simulink model "distributed_project_square"  (R2025b)
settings: Solver=VariableStepAuto  StartTime=0.0  StopTime=10  RelTol=1e-3  AbsTol=1e-3  EnableMultiTasking=on
model workspace (MAT data in the model file):
  t_now = 10
  v = 1
values from neighbouring files (symbols this model uses):
  m = 20    [FirstRegression.m]
  msg_init =     [distributed_project_adjusted.mat]
  N = min([length(e1), length(e2), length(e3), N_max])    [10_runs_result_for_odometer.m]    (also in cc.m = min(length(e1), length(e2)); distributed_project_adjusted.mat = 100; distributed_stats.m = min([length(e1),length(e2),length(e3)]); ten_runs_result_for_odometer.m)
  r = 0.05    [distributed_project.mat]    (also in distributed_project_adjusted.mat)
undefined symbols (not defined in the file or in its folder): fractalcoef, X, Y, Z
libraries: nesl_utility x69, sm_lib x50, simulink x20, matrix_library x20, mspfiltlib x4, sensorgpslib x4, mspsensorlib x4
(part 4 of 5)

== matlab function distributed_project_square/MATLAB Function1 ==
  data: x output; lat input; y output; lon input
function [x,y] = getXY(lat, lon)

% Reference point
persistent lat0 lon0 initialized

if isempty(initialized)
    lat0 = lat;
    lon0 = lon;
    initialized = true;
end



% Convert to radians
lat0_rad = deg2rad(lat0);
lon0_rad = deg2rad(lon0);
lat_rad  = deg2rad(lat);
lon_rad  = deg2rad(lon);

% Earth radius
R = 6371000; % meters

% Compute local x, y
lat_avg = (lat_rad + lat0_rad)/2;
x = R * (lon_rad - lon0_rad) * cos(lat_avg); % east
y = R * (lat_rad - lat0_rad);                 % north

== matlab function distributed_project_square/MATLAB Function2 ==
  data: msg_in input; x_hat_neighbors output; neighbor_idx output; P_j_neighbours output; N output; my_id input; t_now input size=1
function [x_hat_neighbors, neighbor_idx, P_j_neighbours, N] = ...
         receive_msg(msg_in, my_id, t_now)
%#codegen

%% Fixed dimensions — must be constants for codegen
MAX_AGENTS  = 7;
STATE_DIM   = 5;
P_DIM       = 5;
T_WINDOW    = 5.0;   % seconds — max message age

N = 0;

for i = 1:length(msg_in)
    if msg_in(i).ID ~= 0   % assume ID=0 means empty slot
        N = N + 1;
    end
end


%% Fixed-size outputs — codegen requires known dimensions
x_hat_neighbors = zeros(STATE_DIM, MAX_AGENTS);
P_j_neighbours  = zeros(P_DIM, P_DIM, MAX_AGENTS);
neighbor_idx    = zeros(1, MAX_AGENTS);
N_neighbors     = 0;




%% Persistent store — holds latest message per agent slot
%% Indexed by agent ID (1..MAX_AGENTS)
persistent latest_x latest_P latest_t latest_valid

if isempty(latest_x)
    latest_x     = zeros(STATE_DIM, MAX_AGENTS);
    latest_P     = zeros(P_DIM, P_DIM, MAX_AGENTS);
    latest_t     = -inf(1, MAX_AGENTS);   % never received
    latest_valid = zeros(1, MAX_AGENTS);  % 0 = no data
end

%% ── Step 1: Update persistent store with incoming messages ────────
for k = 1:length(msg_in)
    id = msg_in(k).ID;

    %% Skip invalid IDs
    if id < 1 || id > N
        continue;
    end

    %% Skip own messages
    if id == my_id
        continue;
    end

    %% Keep only the latest message per ID
    if msg_in(k).t > latest_t(id)
        latest_x(:, id)      = msg_in(k).x;
        latest_P(:, :, id)   = msg_in(k).P;
        latest_t(id)         = msg_in(k).t;
        latest_valid(id)     = 1;
    end
end

%% ── Step 2: Collect valid neighbours within time window ───────────
for id = 1:N

    %% Skip self
    if id == my_id
        continue;
    end

    %% Skip slots never received
    if latest_valid(id) == 0
        continue;
    end

    %% Skip stale messages
    msg_age = t_now - latest_t(id);
    if msg_age > T_WINDOW || msg_age < 0
        continue;
    end

    %% Valid neighbour — add to output
    N_neighbors = N_neighbors + 1;
    x_hat_neighbors(:, N_neighbors) = latest_x(:, id);
    P_j_neighbours(:,:, N_neighbors) = latest_P(:,:, id);
    neighbor_idx(N_neighbors) = id;
end





end

== matlab function distributed_project_square/Subsystem2/MATLAB Function8 ==
  data: N_i input; N_final output; trigger output
function [N_final, trigger] = convergence_detector(N_i)

%#codegen

% PARAMETERS
k = 5;   % number of steps for stability

% PERSISTENT MEMORY
persistent buffer count

    if isempty(buffer)
        buffer = zeros(k,1);
        count = 0;
    end

% SHIFT BUFFER (like Unit Delay chain)
buffer = [buffer(2:end); N_i];

% CHECK IF ALL VALUES SAME


    if all(buffer == buffer(1))
        count = count + 1;
    else
        count = 0;
    end

    % TRIGGER WHEN STABLE
    if count >= 1   % already stable for k steps
        trigger = 1;
        N_final = buffer(end);
    else
        trigger = 0;
        N_final = N_i;
    end

end

== matlab function distributed_project_square/MATLAB Function4 ==
  data: ID_i input; delta_i output double; N input; formation input
function delta_i = formation_calculator(ID_i, N, formation)
    %#codegen
    
    delta_i = [0; 0];
    
    if N <= 0 || ID_i < 1 || ID_i > N || N == 1
        return;
    end
    spacing = 1.5;
    switch formation
        case 1  % LINE (N ≤ 2)
            center = (N - 1) / 2;
            delta_i = double([(ID_i - 1 - center) * spacing; 0]);
            
        case 2  % CIRCLE (N ≥ 5)
            radius = spacing * N / (2 * pi);
            theta = 2 * pi * (ID_i - 1) / N;
            delta_i = radius * [cos(double(theta)); sin(double(theta))];
            
        case 3  % SQUARE (N = 4)
            half = spacing / 2;
            corners = [ half, -half, -half,  half;   % x-coordinates
                       -half, -half,  half,  half];  % y-coordinates
            delta_i = corners(:, ID_i);
            
        case 4  % TRIANGLE (N = 3)
            side = spacing * 2;
            h = sqrt(3) / 2 * side;
            vertices = [0,   -side/2,  side/2;    % x-coordinates
                       2*h/3, -h/3,   -h/3];     % y-coordinates
            delta_i = vertices(:, ID_i);
            
        otherwise
            delta_i = [0; 0];
    end
end

== matlab function distributed_project_square/MATLAB Function5 ==
  data: N_final input; formation output
function formation = formation_selector(N_final)


    if N_final <= 0
        formation = 0;  % Invalid
        warning('Invalid number of agents: %d', N_final);
        return;
    end

    if N_final <= 2
        formation = 1;
    elseif N_final == 3
        formation = 4;
    elseif N_final == 4
        formation = 3;
    else
        formation = 2;
    end

end

== matlab function distributed_project_square/MATLAB Function6 ==
  data: x_fused input; ei_pos_f output; x_c input; delta_i input; ei_norm output; x_c_raw input
function [ei_pos_f, ei_norm] = formation_error_calculator(...
                               x_fused, x_c, delta_i, x_c_raw)
%#codegen
persistent ei_prev;
if isempty(ei_prev)
    ei_prev = zeros(2,1);
end
ei_pos_raw = (x_c + delta_i) - x_fused(1:2);

%% Low-pass filter — smooth noise
alpha    = 0.167;   % Ts=0.01, tau=0.05s
ei_pos_f = (1-alpha)*ei_prev + alpha*ei_pos_raw;

%% Use raw norm for threshold (not filtered)
ei_norm = norm((x_c_raw + delta_i) - x_fused(1:2));
ei_prev = ei_pos_f;
end

== matlab function distributed_project_square/MATLAB Function7 ==
  data: ei_pos input; ei_vel input; kp input; kd input; L input; vL output size=1; vR output size=1; theta input; w_scaled output; u output
function [vL, vR, w_scaled, u] = control_law(ei_pos, ei_vel, kp, kd, L, theta)
%#codegen

u = [0.0; 0.0];
w_scaled = double(0);
vL = double(0);
vR = double(0);

%% Deadband for spacing=0.3m
e_dead = 0.08;
if norm(ei_pos) < e_dead
    return;
end

u = kp * ei_pos - kd * ei_vel;

%% Tighter saturation for small formation
u_max  = 0.4;
u_norm = sqrt(u(1)^2 + u(2)^2);
if u_norm > u_max
    u = u * (u_max / u_norm);
end

v_lin =  cos(theta)*u(1) + sin(theta)*u(2);
w     = -sin(theta)*u(1) + cos(theta)*u(2);

w_scaled = w / (L/2);

v_max = 0.4;     % slower for small formation
w_max = 0.4;
v_lin    = max(-v_max, min(v_max, v_lin));
w_scaled = max(-w_max, min(w_max, w_scaled));

vL = v_lin - (L/2)*w_scaled;
vR = v_lin + (L/2)*w_scaled;
end

== matlab function distributed_project_square/Subsystem/MATLAB Function1 ==
  data: pos_x input; x_next output; pos_y input; theta input; v input; a input; w input; P_next output; gyro_bias input
function [x_next, P_next] = local_ekf_predict(pos_x,pos_y, theta, v, a, w, gyro_bias)
% MOTION_UPDATE: Predicts the next state and covariance for a 2D vehicle
%
% Inputs:
%   x  - current state [x; y; theta; v]
%   P  - current state covariance (4x4)
%   u  - control input [a; omega] (acceleration, angular rate)
%   Q  - process noise covariance (4x4)
%   dt - time step Δt
%
% Outputs:
%   x_next - predicted next state
%   P_next - predicted next covariance

dt = 0.01;
Q = eye(5)*0.01;
% Make P persistent across calls
persistent P;
    if isempty(P)
        P = eye(5) * 0.1;  % initialize first time
    end

% State prediction (nonlinear)
x_next = zeros(5,1);

              % angular velocity (yaw)
bias_z = gyro_bias(3);      % gyro bias (yaw)
v = norm(v);
a = norm(a);
x_next(1) = pos_x + v * cos(theta) * dt;
x_next(2) = pos_y + v * sin(theta) * dt;
x_next(3) = theta + w * dt;
x_next(4) = v + a * dt;
x_next(5) = bias_z;

% Jacobian F_k = ∂f/∂x
A = [ 1, 0, -v*sin(theta)*dt, cos(theta)*dt, 0;
      0, 1,  v*cos(theta)*dt, sin(theta)*dt, 0;
      0, 0, 1,                 0,            -dt;
      0, 0, 0,                 1,             0;
      0, 0, 0,                 0,             1];

% Covariance prediction
P_next = A * P * A' + Q;
P = P_next;
end

== matlab function distributed_project_square/MATLAB Function10 ==
  data: quat input; theta output
function theta = quat_to_angle(quat)
%#codegen

% normalize (important if coming from simulation)
quat = quat / norm(quat);

w = quat(1);
z = quat(4);

theta = 2 * atan2(z, w);

end

== matlab function distributed_project_square/MATLAB Function11 ==
  data: x output; lat input; y output; lon input
function [x,y] = getXY(lat, lon)

% Reference point
persistent lat0 lon0 initialized

if isempty(initialized)
    lat0 = lat;
    lon0 = lon;
    initialized = true;
end



% Convert to radians
lat0_rad = deg2rad(lat0);
lon0_rad = deg2rad(lon0);
lat_rad  = deg2rad(lat);
lon_rad  = deg2rad(lon);

% Earth radius
R = 6371000; % meters

% Compute local x, y
lat_avg = (lat_rad + lat0_rad)/2;
x = R * (lon_rad - lon0_rad) * cos(lat_avg); % east
y = R * (lat_rad - lat0_rad);                 % north

== matlab function distributed_project_square/MATLAB Function12 ==
  data: x_c_raw input; x_c_out output size=[2, 1]; all_converged input; x_c_raw output
function [x_c_out, x_c_raw] = centroid_manager(x_c_raw, all_converged)
%#codegen

persistent x_c_latched is_latched;
if isempty(x_c_latched)
    x_c_latched = zeros(2,1);
    is_latched  = false;
end

if all_converged && ~is_latched
    %% Latch centroid at moment of convergence
    x_c_latched = x_c_raw;
    is_latched  = true;
end

if is_latched
    x_c_out = x_c_latched;
else
    x_c_out = x_c_raw;
end
end

== matlab function distributed_project_square/MATLAB Function13 ==
  data: x_i_cons input; x_hat_neighbors input; N_all input; x_c output
function x_c = centroid_estimator(x_i_cons, x_hat_neighbors, N_all)
%#codegen
%% Inputs:
%%   x_i_cons        - own consensus state  (5×1)
%%   x_hat_neighbors - neighbour states     (5×N_neighbors)
%%                     columns 1..N_neighbors are valid
%%   N_neighbors     - actual neighbour count (not N_max)
%%
%% Output:
%%   x_c             - centroid (2×1)

%% Own position — always (2×1) after explicit indexing
own_pos = [x_i_cons(1); x_i_cons(2)];   % explicit 2×1, no reshape


%% Sum own position
pos_sum = own_pos;

%% Add each neighbour position explicitly
for j = 1:N_all-1
    pos_sum = pos_sum + [x_hat_neighbors(1,j); x_hat_neighbors(2,j)];
end

%% Average over total count
x_c   = pos_sum / N_all;
end

== matlab function distributed_project_square/MATLAB Function14 ==
  data: ID_i input; delta_i output double; N input; formation input
function delta_i = formation_calculator(ID_i, N, formation)
    %#codegen
    
    delta_i = [0; 0];
    
    if N <= 0 || ID_i < 1 || ID_i > N || N == 1
        return;
    end
    spacing = 1.5;
    switch formation
        case 1  % LINE (N ≤ 2)
            center = (N - 1) / 2;
            delta_i = double([(ID_i - 1 - center) * spacing; 0]);
            
        case 2  % CIRCLE (N ≥ 5)
            radius = spacing * N / (2 * pi);
            theta = 2 * pi * (ID_i - 1) / N;
            delta_i = radius * [cos(double(theta)); sin(double(theta))];
            
        case 3  % SQUARE (N = 4)
            half = spacing / 2;
            corners = [ half, -half, -half,  half;   % x-coordinates
                       -half, -half,  half,  half];  % y-coordinates
            delta_i = corners(:, ID_i);
            
        case 4  % TRIANGLE (N = 3)
            side = spacing * 2;
            h = sqrt(3) / 2 * side;
            vertices = [0,   -side/2,  side/2;    % x-coordinates
                       2*h/3, -h/3,   -h/3];     % y-coordinates
            delta_i = vertices(:, ID_i);
            
        otherwise
            delta_i = [0; 0];
    end
end

== matlab function distributed_project_square/MATLAB Function15 ==
  data: N_final input; formation output
function formation = formation_selector(N_final)


    if N_final <= 0
        formation = 0;  % Invalid
        warning('Invalid number of agents: %d', N_final);
        return;
    end

    if N_final <= 2
        formation = 1;
    elseif N_final == 3
        formation = 4;
    elseif N_final == 4
        formation = 3;
    else
        formation = 2;
    end

end

== matlab function distributed_project_square/MATLAB Function17 ==
  data: x_fused input; ei_pos_f output; x_c input; delta_i input; ei_norm output; x_c_raw input
function [ei_pos_f, ei_norm] = formation_error_calculator(...
                               x_fused, x_c, delta_i, x_c_raw)
%#codegen
persistent ei_prev;
if isempty(ei_prev)
    ei_prev = zeros(2,1);
end
ei_pos_raw = (x_c + delta_i) - x_fused(1:2);

%% Low-pass filter — smooth noise
alpha    = 0.167;   % Ts=0.01, tau=0.05s
ei_pos_f = (1-alpha)*ei_prev + alpha*ei_pos_raw;

%% Use raw norm for threshold (not filtered)
ei_norm = norm((x_c_raw + delta_i) - x_fused(1:2));
ei_prev = ei_pos_f;
end

== matlab function distributed_project_square/MATLAB Function18 ==
  data: ei_pos input; ei_vel input; kp input; kd input; L input; vL output size=1; vR output size=1; theta input; w_scaled output; u output
function [vL, vR, w_scaled, u] = control_law(ei_pos, ei_vel, kp, kd, L, theta)
%#codegen

u = [0.0; 0.0];
w_scaled = double(0);
vL = double(0);
vR = double(0);

%% Deadband for spacing=0.3m
e_dead = 0.08;
if norm(ei_pos) < e_dead
    return;
end

u = kp * ei_pos - kd * ei_vel;

%% Tighter saturation for small formation
u_max  = 0.4;
u_norm = sqrt(u(1)^2 + u(2)^2);
if u_norm > u_max
    u = u * (u_max / u_norm);
end

v_lin =  cos(theta)*u(1) + sin(theta)*u(2);
w     = -sin(theta)*u(1) + cos(theta)*u(2);

w_scaled = w / (L/2);

v_max = 0.4;     % slower for small formation
w_max = 0.4;
v_lin    = max(-v_max, min(v_max, v_lin));
w_scaled = max(-w_max, min(w_max, w_scaled));

vL = v_lin - (L/2)*w_scaled;
vR = v_lin + (L/2)*w_scaled;
end

== matlab function distributed_project_square/MATLAB Function8 ==
  data: ID_i input int32; msg output Bus: msgBus; x_i input; P_i input; t_now input
function msg = create_msg(ID_i, x_i, P_i, t_now)
%#codegen

% Create bus-compatible struct

msg = struct( ...
    'ID', int32(0), ...
    'x',  zeros(size(x_i)), ...
    'P',  zeros(size(P_i)), ...
    't',  0);

% Assign values
msg.ID = ID_i;
msg.x  = x_i;
msg.P  = P_i;
msg.t  = t_now;

end

== matlab function distributed_project_square/MATLAB Function9 ==
  data: msg_in input; x_hat_neighbors output; neighbor_idx output; P_j_neighbours output; N output; my_id input; t_now input size=1
function [x_hat_neighbors, neighbor_idx, P_j_neighbours, N] = ...
         receive_msg(msg_in, my_id, t_now)
%#codegen

%% Fixed dimensions — must be constants for codegen
MAX_AGENTS  = 7;
STATE_DIM   = 5;
P_DIM       = 5;
T_WINDOW    = 5.0;   % seconds — max message age

N = 0;

for i = 1:length(msg_in)
    if msg_in(i).ID ~= 0   % assume ID=0 means empty slot
        N = N + 1;
    end
end


%% Fixed-size outputs — codegen requires known dimensions
x_hat_neighbors = zeros(STATE_DIM, MAX_AGENTS);
P_j_neighbours  = zeros(P_DIM, P_DIM, MAX_AGENTS);
neighbor_idx    = zeros(1, MAX_AGENTS);
N_neighbors     = 0;




%% Persistent store — holds latest message per agent slot
%% Indexed by agent ID (1..MAX_AGENTS)
persistent latest_x latest_P latest_t latest_valid

if isempty(latest_x)
    latest_x     = zeros(STATE_DIM, MAX_AGENTS);
    latest_P     = zeros(P_DIM, P_DIM, MAX_AGENTS);
    latest_t     = -inf(1, MAX_AGENTS);   % never received
    latest_valid = zeros(1, MAX_AGENTS);  % 0 = no data
end

%% ── Step 1: Update persistent store with incoming messages ────────
for k = 1:length(msg_in)
    id = msg_in(k).ID;

    %% Skip invalid IDs
    if id < 1 || id > N
        continue;
    end

    %% Skip own messages
    if id == my_id
        continue;
    end

    %% Keep only the latest message per ID
    if msg_in(k).t > latest_t(id)
        latest_x(:, id)      = msg_in(k).x;
        latest_P(:, :, id)   = msg_in(k).P;
        latest_t(id)         = msg_in(k).t;
        latest_valid(id)     = 1;
    end
end

%% ── Step 2: Collect valid neighbours within time window ───────────
for id = 1:N

    %% Skip self
    if id == my_id
        continue;
    end

    %% Skip slots never received
    if latest_valid(id) == 0
        continue;
    end

    %% Skip stale messages
    msg_age = t_now - latest_t(id);
    if msg_age > T_WINDOW || msg_age < 0
        continue;
    end

    %% Valid neighbour — add to output
    N_neighbors = N_neighbors + 1;
    x_hat_neighbors(:, N_neighbors) = latest_x(:, id);
    P_j_neighbours(:,:, N_neighbors) = latest_P(:,:, id);
    neighbor_idx(N_neighbors) = id;
end





end

== matlab function distributed_project_square/Subsystem3/MATLAB Function1 ==
  data: pos_x input; x_next output; pos_y input; theta input; v input; a input; w input; P_next output; gyro_bias input
function [x_next, P_next] = local_ekf_predict(pos_x,pos_y, theta, v, a, w, gyro_bias)
% MOTION_UPDATE: Predicts the next state and covariance for a 2D vehicle
%
% Inputs:
%   x  - current state [x; y; theta; v]
%   P  - current state covariance (4x4)
%   u  - control input [a; omega] (acceleration, angular rate)
%   Q  - process noise covariance (4x4)
%   dt - time step Δt
%
% Outputs:
%   x_next - predicted next state
%   P_next - predicted next covariance

dt = 0.01;
Q = eye(5)*0.01;
% Make P persistent across calls
persistent P;
    if isempty(P)
        P = eye(5) * 0.1;  % initialize first time
    end

% State prediction (nonlinear)
x_next = zeros(5,1);

              % angular velocity (yaw)
bias_z = gyro_bias(3);      % gyro bias (yaw)
v = norm(v);
a = norm(a);
x_next(1) = pos_x + v * cos(theta) * dt;
x_next(2) = pos_y + v * sin(theta) * dt;
x_next(3) = theta + w * dt;
x_next(4) = v + a * dt;
x_next(5) = bias_z;

% Jacobian F_k = ∂f/∂x
A = [ 1, 0, -v*sin(theta)*dt, cos(theta)*dt, 0;
      0, 1,  v*cos(theta)*dt, sin(theta)*dt, 0;
      0, 0, 1,                 0,            -dt;
      0, 0, 0,                 1,             0;
      0, 0, 0,                 0,             1];

% Covariance prediction
P_next = A * P * A' + Q;
P = P_next;
end

== matlab function distributed_project_square/Subsystem3/MATLAB Function2 ==
  data: x_bar input; x_hat output; P_bar input; z_actual input; R input; H input; P_hat output
function [x_hat, P_hat] = local_ekf_update(x_bar, P_bar, z_actual, R, H)
% EKF_UPDATE: Performs the measurement update step of an EKF
%
% Inputs:
%   x_bar - predicted state (from motion model)
%   P_bar - predicted covariance (from motion model)
%   z     - measurement vector
%   R     - measurement noise covariance
%   h     - function handle for measurement model h(x)
%   H_    - Jacobian H = dh/dx at x_bar
%
% Outputs:
%   x_hat - updated state estimate
%   P_hat - updated covariance estimate

% 1. Compute predicted measurement
% Measurement function evaluated at x
h = [ ...
    x_bar(1);  % gps_x
    x_bar(2);  % gps_y
    x_bar(3);  % imu_theta
    x_bar(4);  % v_enc
    x_bar(5)   % gyro_bias
];

% Jacobian
z_pred = h;

% 2. Innovation
y = z_actual - z_pred;

% 4. Innovation covariance
S = H * P_bar * H' + R;
% Check condition number and add regularization if needed
    if rcond(S) < 1e-12
        % Add small diagonal perturbation
        S = S + 1e-6 * eye(size(S));
        warning('S matrix near singular, added regularization');
    end
% 5. Kalman gain
W = (P_bar * H') * pinv(S);

% 6. Update state
x_hat = x_bar + W * y;

% 7. Update covariance
I = eye(length(x_bar));
P_hat = (I - W * H) * P_bar;

end

== matlab function distributed_project_square/Subsystem3/MATLAB Function3 ==
  data: z input; R output
function R = getR(z)
    % Compute measurement noise covariance matrix
    % z: matrix where rows = samples, columns = different sensors
    % Returns: full covariance matrix (including cross-terms)
    
    z_detrended = z - mean(z, 1);  % Remove mean from each column
    R = cov(z_detrended);           % Full covariance matrix
    
end

== matlab function distributed_project_square/Subsystem3/MATLAB Function4 ==
  data: H output; x_ input size=[5 1]
function H = compute_jacobian(x_)
assert(numel(x_) == 5);
% Ensure column vector
x_ = x_(:);



% Measurement function evaluated at x
h = [ ...
    x_(1);  % gps_x
    x_(2);  % gps_y
    x_(3);  % imu_theta
    x_(4);  % v_enc
    x_(5)   % gyro_bias
];

% Jacobian
H = eye(5);

end

== matlab function distributed_project_square/Subsystem3/MATLAB Function5 ==
  data: gps_x input; z_actual output; gps_y input; theta_imu input; v_enc input; w_imu input
function z_actual = get_z(gps_x, gps_y, theta_imu, v_enc, w_imu)
v_enc = norm(v_enc);
z_actual = [gps_x; gps_y; theta_imu; v_enc; w_imu];

== matlab function distributed_project_square/MATLAB Function ==
  data: x output; lat input; y output; lon input
function [x,y] = getXY(lat, lon)

% Reference point
persistent lat0 lon0 initialized

if isempty(initialized)
    lat0 = lat;
    lon0 = lon;
    initialized = true;
end



% Convert to radians
lat0_rad = deg2rad(lat0);
lon0_rad = deg2rad(lon0);
lat_rad  = deg2rad(lat);
lon_rad  = deg2rad(lon);

% Earth radius
R = 6371000; % meters

% Compute local x, y
lat_avg = (lat_rad + lat0_rad)/2;
x = R * (lon_rad - lon0_rad) * cos(lat_avg); % east
y = R * (lat_rad - lat0_rad);                 % north

== matlab function distributed_project_square/Subsystem4/MATLAB Function ==
  data: vR input; vL input; fx output; fy output; vx_actual input; vy_actual input; theta input; w_desired input; tau_z output; w_actual input
function [fx, fy, tau_z] = planar_control(vR, vL, vx_actual, vy_actual, theta, ...
                                  w_desired, w_actual)
%#codegen

% --- linear control (vector form) ---
Kp_pos = 10;

% desired velocity in world frame
v_desired = (vR + vL)/2;
vx_des = v_desired * cos(theta);
vy_des = v_desired * sin(theta);

% force based on velocity error
fx = Kp_pos * (vx_des - vx_actual);
fy = Kp_pos * (vy_des - vy_actual);
%#codegen
%% Simple P controller on angular velocity
%% tau = I * (w_desired - w_actual) / Ts
Kp_heading = 0.3;        % tune this
tau_z = Kp_heading * (w_desired - w_actual);
if vR==0 || vL==0
    tau_z = 0;
    fx = 0;
    fy = 0;
end
%% Torque must be 3x1 for Spherical Primitive (x,y,z torques)
%% Only Z torque for planar rotation
tau = [0; 0; tau_z];
end

== matlab function distributed_project_square/MATLAB Function16 ==
  data: ID_i input int32; msg output Bus: msgBus; x_i input; P_i input; t_now input
function msg = create_msg(ID_i, x_i, P_i, t_now)
%#codegen

% Create bus-compatible struct

msg = struct( ...
    'ID', int32(0), ...
    'x',  zeros(size(x_i)), ...
    'P',  zeros(size(P_i)), ...
    't',  0);

% Assign values
msg.ID = ID_i;
msg.x  = x_i;
msg.P  = P_i;
msg.t  = t_now;

end

== matlab function distributed_project_square/Subsystem4/MATLAB Function1 ==
  data: vL_actual input; v_xyz output; vR_actual input; theta input
function v_xyz = compute_velocity(vL_actual, vR_actual, theta)
%#codegen

v_true = (vL_actual + vR_actual) / 2;
vx = v_true * cos(theta);
vy = v_true * sin(theta);
vz = 0;

v_xyz = [vx; vy; vz];   % 3x1 vector

end

== matlab function distributed_project_square/Subsystem4/MATLAB Function2 ==
  data: vL_actual input; w_true output; vR_actual input; L input
function w_true = compute_angular_velocity(vL_actual, vR_actual, L)
%#codegen

w_true = (vR_actual - vL_actual) / L;

end

== matlab function distributed_project_square/Subsystem4/MATLAB Function24 ==
  data: quat input; theta output
function theta = quat_to_angle(quat)
%#codegen

% normalize (important if coming from simulation)
quat = quat / norm(quat);

w = quat(1);
z = quat(4);

theta = 2 * atan2(z, w);

end

== matlab function distributed_project_square/Subsystem5/MATLAB Function ==
  data: N input; neighbour_idx input; x_j_hat output; x_hat_neighbours input; P_j output; P_j_neighbours input
function [x_j_hat, P_j] = neighbour_ekf_update(N, neighbour_idx, x_hat_neighbours, P_j_neighbours)
% EKF_UPDATE: Performs the measurement update step of an EKF
%
% Inputs:
%   x_bar - predicted state (from motion model)
%   P_bar - predicted covariance (from motion model)
%   z     - measurement vector
%   R     - measurement noise covariance
%   h     - function handle for measurement model h(x)
%   H_    - Jacobian H = dh/dx at x_bar
%
% Outputs:
%   x_hat - updated state estimate
%   P_hat - updated covariance estimate

% 1. Compute predicted measurement
state_dim = size(x_hat_neighbours, 1);          % Number of rows
P_dim = size(P_j_neighbours, 1);                % Covariance dimension

% Initialize outputs
x_j_hat = zeros(state_dim, length(neighbour_idx));
P_j = zeros(P_dim, P_dim, length(neighbour_idx));

    for k = 1:N-1
        x_j_bar = x_hat_neighbours(:, k);           % state_dim × 1
        P_j_bar = P_j_neighbours(:, :, k);
    
   
        x_j_bar = x_j_bar(:);
        
        
        
        % Measurement function evaluated at x
        h = [ ...
            x_j_bar(1);  % gps_x
            x_j_bar(2);  % gps_y
            x_j_bar(3);  % imu_theta
            x_j_bar(4);  % v_enc
            x_j_bar(5)   % gyro_bias
        ];
        
        % Jacobian
        H_j = eye(5);
    
    
        z_j = h;
    
        z_detrended = z_j - mean(z_j, 1);  % Remove mean from each column
        R_comm = cov(z_detrended);    
        if rcond(P_j_bar) < 1e-12
            % Add small diagonal perturbation
            P_j_bar = P_j_bar + 1e-6 * eye(size(P_j_bar));
            warning('P_j_bar matrix near singular, added regularization');
        end

        if rcond(R_comm) < 1e-12
            % Add small diagonal perturbation
            R_comm = R_comm + 1e-6 * eye(size(R_comm));
            warning('R_comm matrix near singular, added regularization');
        end
        % 5. Kalman gain
        temp = (P_j_bar + R_comm);
        W_j = P_j_bar * pinv(temp) ;
        
        % 6. Update state
        x_j_hat(:,k) = x_j_bar + W_j * (z_j - x_j_bar);
       
        % 7. Update covariance
        I = eye(state_dim);
        P_j(:,:, k) = (I - W_j * H_j) * P_j_bar;
    
    end
end

== matlab function distributed_project_square/Subsystem5/MATLAB Function1 ==
  data: x_i_hat input; x_fused output; P_i input; P_j input; x_j_hat input; P_fused output; N_j input
function [x_fused, P_fused] = information_fusion(x_i_hat, P_i, P_j, x_j_hat, N_j)
% EKF_UPDATE: Performs the measurement update step of an EKF
%
% Inputs:
%   x_bar - predicted state (from motion model)
%   P_bar - predicted covariance (from motion model)
%   z     - measurement vector
%   R     - measurement noise covariance
%   h     - function handle for measurement model h(x)
%   H_    - Jacobian H = dh/dx at x_bar
%
% Outputs:
%   x_hat - updated state estimate
%   P_hat - updated covariance estimate

% 1. Compute predicted measurement

P_fused = P_i;
x_fused = x_i_hat;

    for j = 1:N_j-1
        P_prev = P_fused;
        x_prev = x_fused;
        if rcond(P_prev) < 1e-12
            % Add small diagonal perturbation
            P_prev = P_prev + 1e-6 * eye(size(P_prev));
            warning('P_prev matrix near singular, added regularization');
        end
            
        if rcond(P_j(:,:,j)) < 1e-12
            % Add small diagonal perturbation
            P_j(:,:,j) = P_j(:,:,j) + 1e-6 * eye(size(P_j(:,:,j)));
            warning('P_j matrix near singular, added regularization');
        end
        % 5. Kalman gain
        temp = (trace(pinv(P_prev)) + trace(pinv(P_j(:,:,j))));
      
        alpha = trace(pinv(P_prev)) * pinv(temp) ;
        P_fused_inv = alpha*pinv(P_prev) + (1-alpha)*pinv(P_j(:,:,j));
        P_fused = pinv(P_fused_inv);
        x_fused = P_fused * (alpha*pinv(P_prev)*x_prev + (1-alpha)*pinv(P_j(:,:,j))*x_j_hat(:,j));
    end


end

== matlab function distributed_project_square/Subsystem5/MATLAB Function2 ==
  data: x_i_hat input; x_i_cons output; x_hat_neighbors input; N input
function x_i_cons  = consensus_update(x_i_hat, x_hat_neighbors,N)
% CONSENSUS_BLOCK - Multi-agent consensus update
%
% Inputs:
%   x_hat_i         - current state estimate of agent i (scalar or vector)
%   x_hat_neighbors - matrix of neighbor estimates (each column = neighbor)
%   a_ij            - vector of weights for each neighbor
%   gain            - epsilon (continuous) or gamma (discrete)
%   dt              - timestep (for discrete integration if mode='continuous')
%   mode            - 'continuous' or 'discrete'
%
% Output:
%   x_hat_next      - updated state estimate of agent i

% Compute weighted difference with neighbors
gamma = 0.05;
N_neighbours = size(x_hat_neighbors, 2); 
a_ij = zeros(1:N_neighbours);
x_i_cons = zeros(size(x_i_hat));
% number of neighbors
a_ij(:) = 1/N_neighbours;  
diff = zeros(size(x_i_hat));
    for j = 1:N-1
        diff = diff + a_ij(j) * (x_hat_neighbors(:,j) - x_i_hat);
            
    end
x_i_cons = x_i_hat + gamma * diff;

end

== matlab function distributed_project_square/Subsystem/MATLAB Function2 ==
  data: x_bar input; x_hat output; P_bar input; z_actual input; R input; H input; P_hat output
function [x_hat, P_hat] = local_ekf_update(x_bar, P_bar, z_actual, R, H)
% EKF_UPDATE: Performs the measurement update step of an EKF
%
% Inputs:
%   x_bar - predicted state (from motion model)
%   P_bar - predicted covariance (from motion model)
%   z     - measurement vector
%   R     - measurement noise covariance
%   h     - function handle for measurement model h(x)
%   H_    - Jacobian H = dh/dx at x_bar
%
% Outputs:
%   x_hat - updated state estimate
%   P_hat - updated covariance estimate

% 1. Compute predicted measurement
% Measurement function evaluated at x
h = [ ...
    x_bar(1);  % gps_x
    x_bar(2);  % gps_y
    x_bar(3);  % imu_theta
    x_bar(4);  % v_enc
    x_bar(5)   % gyro_bias
];

% Jacobian
z_pred = h;

% 2. Innovation
y = z_actual - z_pred;

% 4. Innovation covariance
S = H * P_bar * H' + R;
% Check condition number and add regularization if needed
    if rcond(S) < 1e-12
        % Add small diagonal perturbation
        S = S + 1e-6 * eye(size(S));
        warning('S matrix near singular, added regularization');
    end
% 5. Kalman gain
W = (P_bar * H') * pinv(S);

% 6. Update state
x_hat = x_bar + W * y;

% 7. Update covariance
I = eye(length(x_bar));
P_hat = (I - W * H) * P_bar;

end

== matlab function distributed_project_square/MATLAB Function19 ==
  data: x output; lat input; y output; lon input
function [x,y] = getXY(lat, lon)

% Reference point
persistent lat0 lon0 initialized

if isempty(initialized)
    lat0 = lat;
    lon0 = lon;
    initialized = true;
end



% Convert to radians
lat0_rad = deg2rad(lat0);
lon0_rad = deg2rad(lon0);
lat_rad  = deg2rad(lat);
lon_rad  = deg2rad(lon);

% Earth radius
R = 6371000; % meters

% Compute local x, y
lat_avg = (lat_rad + lat0_rad)/2;
x = R * (lon_rad - lon0_rad) * cos(lat_avg); % east
y = R * (lat_rad - lat0_rad);                 % north

== matlab function distributed_project_square/MATLAB Function20 ==
  data: ID_i input int32; msg output Bus: msgBus; x_i input; P_i input; t_now input
function msg = create_msg(ID_i, x_i, P_i, t_now)
%#codegen

% Create bus-compatible struct

msg = struct( ...
    'ID', int32(0), ...
    'x',  zeros(size(x_i)), ...
    'P',  zeros(size(P_i)), ...
    't',  0);

% Assign values
msg.ID = ID_i;
msg.x  = x_i;
msg.P  = P_i;
msg.t  = t_now;

end

== matlab function distributed_project_square/MATLAB Function21 ==
  data: msg_in input; x_hat_neighbors output; neighbor_idx output; P_j_neighbours output; N output; my_id input; t_now input size=1
function [x_hat_neighbors, neighbor_idx, P_j_neighbours, N] = ...
         receive_msg(msg_in, my_id, t_now)
%#codegen

%% Fixed dimensions — must be constants for codegen
MAX_AGENTS  = 7;
STATE_DIM   = 5;
P_DIM       = 5;
T_WINDOW    = 5.0;   % seconds — max message age

N = 0;

for i = 1:length(msg_in)
    if msg_in(i).ID ~= 0   % assume ID=0 means empty slot
        N = N + 1;
    end
end


%% Fixed-size outputs — codegen requires known dimensions
x_hat_neighbors = zeros(STATE_DIM, MAX_AGENTS);
P_j_neighbours  = zeros(P_DIM, P_DIM, MAX_AGENTS);
neighbor_idx    = zeros(1, MAX_AGENTS);
N_neighbors     = 0;




%% Persistent store — holds latest message per agent slot
%% Indexed by agent ID (1..MAX_AGENTS)
persistent latest_x latest_P latest_t latest_valid

if isempty(latest_x)
    latest_x     = zeros(STATE_DIM, MAX_AGENTS);
    latest_P     = zeros(P_DIM, P_DIM, MAX_AGENTS);
    latest_t     = -inf(1, MAX_AGENTS);   % never received
    latest_valid = zeros(1, MAX_AGENTS);  % 0 = no data
end

%% ── Step 1: Update persistent store with incoming messages ────────
for k = 1:length(msg_in)
    id = msg_in(k).ID;

    %% Skip invalid IDs
    if id < 1 || id > N
        continue;
    end

    %% Skip own messages
    if id == my_id
        continue;
    end

    %% Keep only the latest message per ID
    if msg_in(k).t > latest_t(id)
        latest_x(:, id)      = msg_in(k).x;
        latest_P(:, :, id)   = msg_in(k).P;
        latest_t(id)         = msg_in(k).t;
        latest_valid(id)     = 1;
    end
end

%% ── Step 2: Collect valid neighbours within time window ───────────
for id = 1:N

    %% Skip self
    if id == my_id
        continue;
    end

    %% Skip slots never received
    if latest_valid(id) == 0
        continue;
    end

    %% Skip stale messages
    msg_age = t_now - latest_t(id);
    if msg_age > T_WINDOW || msg_age < 0
        continue;
    end

    %% Valid neighbour — add to output
    N_neighbors = N_neighbors + 1;
    x_hat_neighbors(:, N_neighbors) = latest_x(:, id);
    P_j_neighbours(:,:, N_neighbors) = latest_P(:,:, id);
    neighbor_idx(N_neighbors) = id;
end





end

== matlab function distributed_project_square/MATLAB Function22 ==
  data: quat input; theta output
function theta = quat_to_angle(quat)
%#codegen

% normalize (important if coming from simulation)
quat = quat / norm(quat);

w = quat(1);
z = quat(4);

theta = 2 * atan2(z, w);

end

== matlab function distributed_project_square/MATLAB Function23 ==
  data: quat input; theta output
function theta = quat_to_angle(quat)
%#codegen

% normalize (important if coming from simulation)
quat = quat / norm(quat);

w = quat(1);
z = quat(4);

theta = 2 * atan2(z, w);

end

== matlab function distributed_project_square/MATLAB Function25 ==
  data: x_c_raw input; x_c_out output size=[2, 1]; all_converged input; x_c_raw output
function [x_c_out, x_c_raw] = centroid_manager(x_c_raw, all_converged)
%#codegen

persistent x_c_latched is_latched;
if isempty(x_c_latched)
    x_c_latched = zeros(2,1);
    is_latched  = false;
end

if all_converged && ~is_latched
    %% Latch centroid at moment of convergence
    x_c_latched = x_c_raw;
    is_latched  = true;
end

if is_latched
    x_c_out = x_c_latched;
else
    x_c_out = x_c_raw;
end
end

== matlab function distributed_project_square/MATLAB Function26 ==
  data: x_i_cons input; x_hat_neighbors input; N_all input; x_c output
function x_c = centroid_estimator(x_i_cons, x_hat_neighbors, N_all)
%#codegen
%% Inputs:
%%   x_i_cons        - own consensus state  (5×1)
%%   x_hat_neighbors - neighbour states     (5×N_neighbors)
%%                     columns 1..N_neighbors are valid
%%   N_neighbors     - actual neighbour count (not N_max)
%%
%% Output:
%%   x_c             - centroid (2×1)

%% Own position — always (2×1) after explicit indexing
own_pos = [x_i_cons(1); x_i_cons(2)];   % explicit 2×1, no reshape


%% Sum own position
pos_sum = own_pos;

%% Add each neighbour position explicitly
for j = 1:N_all-1
    pos_sum = pos_sum + [x_hat_neighbors(1,j); x_hat_neighbors(2,j)];
end

%% Average over total count
x_c   = pos_sum / N_all;
end

== matlab function distributed_project_square/MATLAB Function29 ==
  data: ID_i input; delta_i output double; N input; formation input
function delta_i = formation_calculator(ID_i, N, formation)
    %#codegen
    
    delta_i = [0; 0];
    
    if N <= 0 || ID_i < 1 || ID_i > N || N == 1
        return;
    end
    spacing = 1.5;
    switch formation
        case 1  % LINE (N ≤ 2)
            center = (N - 1) / 2;
            delta_i = double([(ID_i - 1 - center) * spacing; 0]);
            
        case 2  % CIRCLE (N ≥ 5)
            radius = spacing * N / (2 * pi);
            theta = 2 * pi * (ID_i - 1) / N;
            delta_i = radius * [cos(double(theta)); sin(double(theta))];
            
        case 3  % SQUARE (N = 4)
            half = spacing / 2;
            corners = [ half, -half, -half,  half;   % x-coordinates
                       -half, -half,  half,  half];  % y-coordinates
            delta_i = corners(:, ID_i);
            
        case 4  % TRIANGLE (N = 3)
            side = spacing * 2;
            h = sqrt(3) / 2 * side;
            vertices = [0,   -side/2,  side/2;    % x-coordinates
                       2*h/3, -h/3,   -h/3];     % y-coordinates
            delta_i = vertices(:, ID_i);
            
        otherwise
            delta_i = [0; 0];
    end
end

== matlab function distributed_project_square/MATLAB Function30 ==
  data: N_final input; formation output
function formation = formation_selector(N_final)


    if N_final <= 0
        formation = 0;  % Invalid
        warning('Invalid number of agents: %d', N_final);
        return;
    end

    if N_final <= 2
        formation = 1;
    elseif N_final == 3
        formation = 4;
    elseif N_final == 4
        formation = 3;
    else
        formation = 2;
    end

end

== matlab function distributed_project_square/MATLAB Function24 ==
  data: quat input; theta output
function theta = quat_to_angle(quat)
%#codegen

% normalize (important if coming from simulation)
quat = quat / norm(quat);

w = quat(1);
z = quat(4);

theta = 2 * atan2(z, w);

end

== matlab function distributed_project_square/Subsystem1/MATLAB Function1 ==
  data: vL_actual input; v_xyz output; vR_actual input; theta input
function v_xyz = compute_velocity(vL_actual, vR_actual, theta)
%#codegen

v_true = (vL_actual + vR_actual) / 2;
vx = v_true * cos(theta);
vy = v_true * sin(theta);
vz = 0;

v_xyz = [vx; vy; vz];   % 3x1 vector

end

== matlab function distributed_project_square/Subsystem1/MATLAB Function2 ==
  data: vL_actual input; w_true output; vR_actual input; L input
function w_true = compute_angular_velocity(vL_actual, vR_actual, L)
%#codegen

w_true = (vR_actual - vL_actual) / L;

end

== matlab function distributed_project_square/MATLAB Function31 ==
  data: x_fused input; ei_pos_f output; x_c input; delta_i input; ei_norm output; x_c_raw input
function [ei_pos_f, ei_norm] = formation_error_calculator(...
                               x_fused, x_c, delta_i, x_c_raw)
%#codegen
persistent ei_prev;
if isempty(ei_prev)
    ei_prev = zeros(2,1);
end
ei_pos_raw = (x_c + delta_i) - x_fused(1:2);

%% Low-pass filter — smooth noise
alpha    = 0.167;   % Ts=0.01, tau=0.05s
ei_pos_f = (1-alpha)*ei_prev + alpha*ei_pos_raw;

%% Use raw norm for threshold (not filtered)
ei_norm = norm((x_c_raw + delta_i) - x_fused(1:2));
ei_prev = ei_pos_f;
end

== matlab function distributed_project_square/MATLAB Function32 ==
  data: ei_pos input; ei_vel input; kp input; kd input; L input; vL output size=1; vR output size=1; theta input; w_scaled output; u output
function [vL, vR, w_scaled, u] = control_law(ei_pos, ei_vel, kp, kd, L, theta)
%#codegen

u = [0.0; 0.0];
w_scaled = double(0);
vL = double(0);
vR = double(0);

%% Deadband for spacing=0.3m
e_dead = 0.08;
if norm(ei_pos) < e_dead
    return;
end

u = kp * ei_pos - kd * ei_vel;

%% Tighter saturation for small formation
u_max  = 0.4;
u_norm = sqrt(u(1)^2 + u(2)^2);
if u_norm > u_max
    u = u * (u_max / u_norm);
end

v_lin =  cos(theta)*u(1) + sin(theta)*u(2);
w     = -sin(theta)*u(1) + cos(theta)*u(2);

w_scaled = w / (L/2);

v_max = 0.4;     % slower for small formation
w_max = 0.4;
v_lin    = max(-v_max, min(v_max, v_lin));
w_scaled = max(-w_max, min(w_max, w_scaled));

vL = v_lin - (L/2)*w_scaled;
vR = v_lin + (L/2)*w_scaled;
end

== matlab function distributed_project_square/Subsystem/MATLAB Function3 ==
  data: z input; R output
function R = getR(z)
    % Compute measurement noise covariance matrix
    % z: matrix where rows = samples, columns = different sensors
    % Returns: full covariance matrix (including cross-terms)
    
    z_detrended = z - mean(z, 1);  % Remove mean from each column
    R = cov(z_detrended);           % Full covariance matrix
    
end

== matlab function distributed_project_square/Subsystem6/MATLAB Function1 ==
  data: pos_x input; x_next output; pos_y input; theta input; v input; a input; w input; P_next output; gyro_bias input
function [x_next, P_next] = local_ekf_predict(pos_x,pos_y, theta, v, a, w, gyro_bias)
% MOTION_UPDATE: Predicts the next state and covariance for a 2D vehicle
%
% Inputs:
%   x  - current state [x; y; theta; v]
%   P  - current state covariance (4x4)
%   u  - control input [a; omega] (acceleration, angular rate)
%   Q  - process noise covariance (4x4)
%   dt - time step Δt
%
% Outputs:
%   x_next - predicted next state
%   P_next - predicted next covariance

dt = 0.01;
Q = eye(5)*0.01;
% Make P persistent across calls
persistent P;
    if isempty(P)
        P = eye(5) * 0.1;  % initialize first time
    end

% State prediction (nonlinear)
x_next = zeros(5,1);

              % angular velocity (yaw)
bias_z = gyro_bias(3);      % gyro bias (yaw)
v = norm(v);
a = norm(a);
x_next(1) = pos_x + v * cos(theta) * dt;
x_next(2) = pos_y + v * sin(theta) * dt;
x_next(3) = theta + w * dt;
x_next(4) = v + a * dt;
x_next(5) = bias_z;

% Jacobian F_k = ∂f/∂x
A = [ 1, 0, -v*sin(theta)*dt, cos(theta)*dt, 0;
      0, 1,  v*cos(theta)*dt, sin(theta)*dt, 0;
      0, 0, 1,                 0,            -dt;
      0, 0, 0,                 1,             0;
      0, 0, 0,                 0,             1];

% Covariance prediction
P_next = A * P * A' + Q;
P = P_next;
end

== matlab function distributed_project_square/Subsystem6/MATLAB Function2 ==
  data: x_bar input; x_hat output; P_bar input; z_actual input; R input; H input; P_hat output
function [x_hat, P_hat] = local_ekf_update(x_bar, P_bar, z_actual, R, H)
% EKF_UPDATE: Performs the measurement update step of an EKF
%
% Inputs:
%   x_bar - predicted state (from motion model)
%   P_bar - predicted covariance (from motion model)
%   z     - measurement vector
%   R     - measurement noise covariance
%   h     - function handle for measurement model h(x)
%   H_    - Jacobian H = dh/dx at x_bar
%
% Outputs:
%   x_hat - updated state estimate
%   P_hat - updated covariance estimate

% 1. Compute predicted measurement
% Measurement function evaluated at x
h = [ ...
    x_bar(1);  % gps_x
    x_bar(2);  % gps_y
    x_bar(3);  % imu_theta
    x_bar(4);  % v_enc
    x_bar(5)   % gyro_bias
];

% Jacobian
z_pred = h;

% 2. Innovation
y = z_actual - z_pred;

% 4. Innovation covariance
S = H * P_bar * H' + R;
% Check condition number and add regularization if needed
    if rcond(S) < 1e-12
        % Add small diagonal perturbation
        S = S + 1e-6 * eye(size(S));
        warning('S matrix near singular, added regularization');
    end
% 5. Kalman gain
W = (P_bar * H') * pinv(S);

% 6. Update state
x_hat = x_bar + W * y;

% 7. Update covariance
I = eye(length(x_bar));
P_hat = (I - W * H) * P_bar;

end

== matlab function distributed_project_square/Subsystem6/MATLAB Function3 ==
  data: z input; R output
function R = getR(z)
    % Compute measurement noise covariance matrix
    % z: matrix where rows = samples, columns = different sensors
    % Returns: full covariance matrix (including cross-terms)
    
    z_detrended = z - mean(z, 1);  % Remove mean from each column
    R = cov(z_detrended);           % Full covariance matrix
    
end

== matlab function distributed_project_square/Subsystem6/MATLAB Function4 ==
  data: H output; x_ input size=[5 1]
function H = compute_jacobian(x_)
assert(numel(x_) == 5);
% Ensure column vector
x_ = x_(:);



% Measurement function evaluated at x
h = [ ...
    x_(1);  % gps_x
    x_(2);  % gps_y
    x_(3);  % imu_theta
    x_(4);  % v_enc
    x_(5)   % gyro_bias
];

% Jacobian
H = eye(5);

end

== matlab function distributed_project_square/Subsystem1/MATLAB Function ==
  data: vR input; vL input; fx output; fy output; vx_actual input; vy_actual input; theta input; w_desired input; tau_z output; w_actual input
function [fx, fy, tau_z] = planar_control(vR, vL, vx_actual, vy_actual, theta, ...
                                  w_desired, w_actual)
%#codegen

% --- linear control (vector form) ---
Kp_pos = 10;

% desired velocity in world frame
v_desired = (vR + vL)/2;
vx_des = v_desired * cos(theta);
vy_des = v_desired * sin(theta);

% force based on velocity error
fx = Kp_pos * (vx_des - vx_actual);
fy = Kp_pos * (vy_des - vy_actual);
%#codegen
%% Simple P controller on angular velocity
%% tau = I * (w_desired - w_actual) / Ts
Kp_heading = 0.3;        % tune this
tau_z = Kp_heading * (w_desired - w_actual);
if vR==0 || vL==0
    tau_z = 0;
    fx = 0;
    fy = 0;
end
%% Torque must be 3x1 for Spherical Primitive (x,y,z torques)
%% Only Z torque for planar rotation
tau = [0; 0; tau_z];
end

== matlab function distributed_project_square/Subsystem1/MATLAB Function24 ==
  data: quat input; theta output
function theta = quat_to_angle(quat)
%#codegen

% normalize (important if coming from simulation)
quat = quat / norm(quat);

w = quat(1);
z = quat(4);

theta = 2 * atan2(z, w);

end

== matlab function distributed_project_square/Subsystem/MATLAB Function4 ==
  data: H output; x_ input size=[5 1]
function H = compute_jacobian(x_)
assert(numel(x_) == 5);
% Ensure column vector
x_ = x_(:);



% Measurement function evaluated at x
h = [ ...
    x_(1);  % gps_x
    x_(2);  % gps_y
    x_(3);  % imu_theta
    x_(4);  % v_enc
    x_(5)   % gyro_bias
];

% Jacobian
H = eye(5);

end

== matlab function distributed_project_square/Subsystem6/MATLAB Function5 ==
  data: gps_x input; z_actual output; gps_y input; theta_imu input; v_enc input; w_imu input
function z_actual = get_z(gps_x, gps_y, theta_imu, v_enc, w_imu)
v_enc = norm(v_enc);
z_actual = [gps_x; gps_y; theta_imu; v_enc; w_imu];

== matlab function distributed_project_square/Subsystem8/MATLAB Function ==
  data: vR input; vL input; fx output; fy output; vx_actual input; vy_actual input; theta input; w_desired input; tau_z output; w_actual input
function [fx, fy, tau_z] = planar_control(vR, vL, vx_actual, vy_actual, theta, ...
                                  w_desired, w_actual)
%#codegen

% --- linear control (vector form) ---
Kp_pos = 10;

% desired velocity in world frame
v_desired = (vR + vL)/2;
vx_des = v_desired * cos(theta);
vy_des = v_desired * sin(theta);

% force based on velocity error
fx = Kp_pos * (vx_des - vx_actual);
fy = Kp_pos * (vy_des - vy_actual);
%#codegen
%% Simple P controller on angular velocity
%% tau = I * (w_desired - w_actual) / Ts
Kp_heading = 0.3;        % tune this
tau_z = Kp_heading * (w_desired - w_actual);
if vR==0 || vL==0
    tau_z = 0;
    fx = 0;
    fy = 0;
end
%% Torque must be 3x1 for Spherical Primitive (x,y,z torques)
%% Only Z torque for planar rotation
tau = [0; 0; tau_z];
end

== matlab function distributed_project_square/Subsystem8/MATLAB Function1 ==
  data: vL_actual input; v_xyz output; vR_actual input; theta input
function v_xyz = compute_velocity(vL_actual, vR_actual, theta)
%#codegen

v_true = (vL_actual + vR_actual) / 2;
vx = v_true * cos(theta);
vy = v_true * sin(theta);
vz = 0;

v_xyz = [vx; vy; vz];   % 3x1 vector

end

== matlab function distributed_project_square/Subsystem8/MATLAB Function2 ==
  data: vL_actual input; w_true output; vR_actual input; L input
function w_true = compute_angular_velocity(vL_actual, vR_actual, L)
%#codegen

w_true = (vR_actual - vL_actual) / L;

end
